simulink model "fourbar"  (Simulink 7.1)
settings: Solver=ode45  StartTime=0.0  StopTime=10  RelTol=1e-3
values from neighbouring files (symbols this model uses):
  m = 0    [FixNode1.m]    (also in FixNode2.m = xy(1,1)-x; SAM.m = str2num(char(m2))-str2num(char(m1)); angle_measurement.m = X(1,2)-X(1,1); m_645.m = 1)
  s = 0    [FixNode2.m]    (also in SAM.m = FixNode2(); linkm.m = -1.57079632679)
libraries: mblibv1 x15
settings Model: Creator=mohsen  LastModifiedBy=mohsen
settings SimMechanicsCC: VisOnUpdateDiagram=on  VisDuringSimulation=on

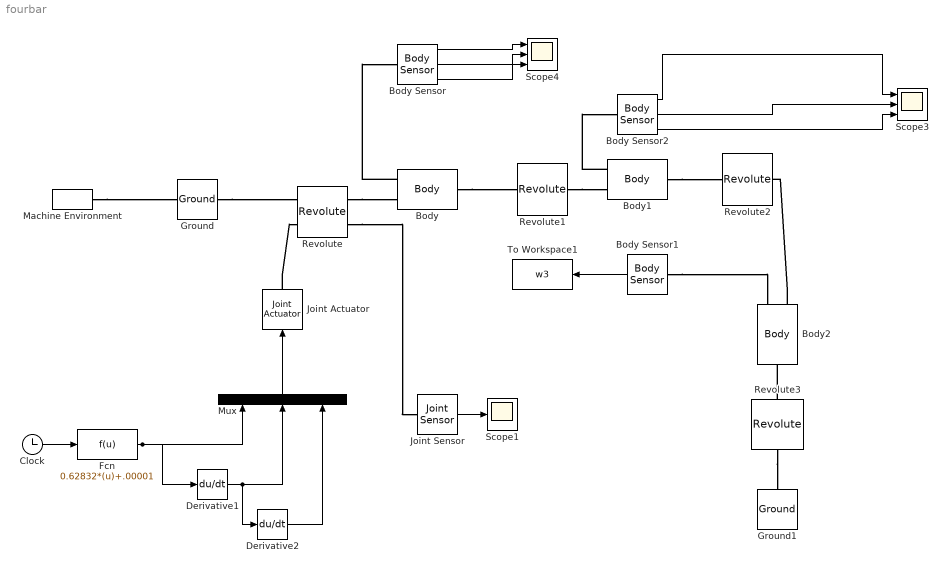
== system fourbar ==
  Body : mblibv1/Bodies/Body  DialogController=MECH.DynMechDlgSource  PhysicalDomain=mechanical  SubClassName=Unknown  LeftPortType=workingframe  RightPortType=workingframe  LConnTagsString=CS3|CS1  RConnTagsString=CS2  DialogClass=MechanicalBodyBlock  Mass=1  MassUnits=kg  InertiaUnits=kg*m^2  Inertia=[.1 0 0;0 .1 0;0 0 .1]  Shape=Cylinder  ShapeDims=[1 1]  ShapeUnits=m  ShapeUse=false  Density=1  DensityUnits=kg/m^3  DensityUse=false  GraphicsMode=1  BodyColor=[0.5 0.5 0.5]  GraphicsObj=[]  AttachedToCS=1  CG=Left$CG$[0 .5 0]$WORLD$WORLD$m$[0 0 0]$Euler X-Y-Z$deg$WORLD$false$none  WorkingFrames=Left$CS3$[0 .5 0]$WORLD$WORLD$m$[0 0 0]$Euler X-Y-Z$deg$WORLD$true$none#Left$CS1$[0 0 0]$World$World$m$[0 0 0]$Euler X-Y-Z$deg$WORLD$true$none#Right$CS2$[0 2 0]$World$World$m$[0 0 0]$Euler X-Y-Z$deg$WORLD$true$none  CGPos=[0 .5 0]  CGRot=[0 0 0]  CS0Pos=[]  CS0Rot=[]  CS1Pos=[0 0 0]  CS1Rot=[0 0 0]  CS2Pos=[0 2 0]  CS2Rot=[0 0 0]  CS3Pos=[0 .5 0]  CS3Rot=[0 0 0]  CS4Pos=[]  CS4Rot=[]  CS5Pos=[]  CS5Rot=[]  CS6Pos=[]  CS6Rot=[]  CS7Pos=[]  CS7Rot=[]  CS8Pos=[]  CS8Rot=[]  CS9Pos=[]  CS9Rot=[]  CS10Pos=[]  CS10Rot=[]  CS11Pos=[]  CS11Rot=[]  CS12Pos=[]  CS12Rot=[]  CS13Pos=[]  CS13Rot=[]  CS14Pos=[]  CS14Rot=[]  CS15Pos=[]  CS15Rot=[]  CS16Pos=[]  CS16Rot=[]  CS17Pos=[]  CS17Rot=[]  CS18Pos=[]  CS18Rot=[]  CS19Pos=[]  CS19Rot=[]  CS20Pos=[]  CS20Rot=[]
  Body Sensor : mblibv1/Sensors &  Actuators/Body Sensor  DialogController=MECH.DynMechDlgSource  SystemSampleTime=-1  PhysicalDomain=Mechanical  PortType=blob  Muxed=off  Pose=off  Angle=on  AngleUnits=deg  ArcVelocity=off  ArcVelocityUnits=deg/s  ArcAcceleration=off  ArcAccelerationUnits=deg/s^2  CoordPosition=on  CoordPositionUnits=m  Velocity=on  VelocityUnits=m/s  Acceleration=on  AccelerationUnits=m/s^2  Quaternion=on  QuaternionDT=off  QuaternionDDT=off  QuaternionUnits=off  OutputVector=[1]  ActiveIO=on  Width=9  DialogClass=MechanicalSensorBlock  ReferenceFrame=Absolute (World)
  Body Sensor1 : mblibv1/Sensors &  Actuators/Body Sensor  Orientation=left  DialogController=MECH.DynMechDlgSource  SystemSampleTime=-1  PhysicalDomain=Mechanical  PortType=blob  Muxed=on  Pose=off  Angle=on  AngleUnits=deg  ArcVelocity=off  ArcVelocityUnits=deg/s  ArcAcceleration=off  ArcAccelerationUnits=deg/s^2  CoordPosition=on  CoordPositionUnits=m  Velocity=off  VelocityUnits=m/s  Acceleration=off  AccelerationUnits=m/s^2  Quaternion=on  QuaternionDT=off  QuaternionDDT=off  QuaternionUnits=off  OutputVector=[1]  ActiveIO=on  Width=3  DialogClass=MechanicalSensorBlock  ReferenceFrame=Absolute (World)
  Body Sensor2 : mblibv1/Sensors &  Actuators/Body Sensor  DialogController=MECH.DynMechDlgSource  SystemSampleTime=-1  PhysicalDomain=Mechanical  PortType=blob  Muxed=off  Pose=off  Angle=on  AngleUnits=deg  ArcVelocity=off  ArcVelocityUnits=deg/s  ArcAcceleration=off  ArcAccelerationUnits=deg/s^2  CoordPosition=on  CoordPositionUnits=m  Velocity=on  VelocityUnits=m/s  Acceleration=on  AccelerationUnits=m/s^2  Quaternion=on  QuaternionDT=off  QuaternionDDT=off  QuaternionUnits=off  OutputVector=[1]  ActiveIO=on  Width=9  DialogClass=MechanicalSensorBlock  ReferenceFrame=Absolute (World)
  Body1 : mblibv1/Bodies/Body  DialogController=MECH.DynMechDlgSource  PhysicalDomain=mechanical  SubClassName=Unknown  LeftPortType=workingframe  RightPortType=workingframe  LConnTagsString=CS3|CS1  RConnTagsString=CS2  DialogClass=MechanicalBodyBlock  Mass=1  MassUnits=kg  InertiaUnits=kg*m^2  Inertia=[.1 0 0;0 .1 0;0 0 .1]  Shape=Cylinder  ShapeDims=[1 1]  ShapeUnits=m  ShapeUse=false  Density=1  DensityUnits=kg/m^3  DensityUse=false  GraphicsMode=1  BodyColor=[0.5 0.5 0.5]  GraphicsObj=[]  AttachedToCS=1  CG=Left$CG$[2 3 0]$WORLD$WORLD$m$[0 0 0]$Euler X-Y-Z$deg$WORLD$false$none  WorkingFrames=Left$CS3$[2 3 0]$WORLD$WORLD$m$[0 0 0]$Euler X-Y-Z$deg$WORLD$true$none#Left$CS1$[0 2 0]$World$World$m$[0 0 0]$Euler X-Y-Z$deg$WORLD$true$none#Right$CS2$[4 4 0]$World$World$m$[0 0 0]$Euler X-Y-Z$deg$WORLD$true$none  CGPos=[2 3 0]  CGRot=[0 0 0]  CS0Pos=[]  CS0Rot=[]  CS1Pos=[0 2 0]  CS1Rot=[0 0 0]  CS2Pos=[4 4 0]  CS2Rot=[0 0 0]  CS3Pos=[2 3 0]  CS3Rot=[0 0 0]  CS4Pos=[]  CS4Rot=[]  CS5Pos=[]  CS5Rot=[]  CS6Pos=[]  CS6Rot=[]  CS7Pos=[]  CS7Rot=[]  CS8Pos=[]  CS8Rot=[]  CS9Pos=[]  CS9Rot=[]  CS10Pos=[]  CS10Rot=[]  CS11Pos=[]  CS11Rot=[]  CS12Pos=[]  CS12Rot=[]  CS13Pos=[]  CS13Rot=[]  CS14Pos=[]  CS14Rot=[]  CS15Pos=[]  CS15Rot=[]  CS16Pos=[]  CS16Rot=[]  CS17Pos=[]  CS17Rot=[]  CS18Pos=[]  CS18Rot=[]  CS19Pos=[]  CS19Rot=[]  CS20Pos=[]  CS20Rot=[]
  Body2 : mblibv1/Bodies/Body  Orientation=down  DialogController=MECH.DynMechDlgSource  PhysicalDomain=mechanical  SubClassName=Unknown  LeftPortType=workingframe  RightPortType=workingframe  LConnTagsString=CS3|CS1  RConnTagsString=CS2  DialogClass=MechanicalBodyBlock  Mass=1  MassUnits=kg  InertiaUnits=kg*m^2  Inertia=[.1 0 0;0 .1 0;0 0 .1]  Shape=Cylinder  ShapeDims=[1 1]  ShapeUnits=m  ShapeUse=false  Density=1  DensityUnits=kg/m^3  DensityUse=false  GraphicsMode=1  BodyColor=[0.5 0.5 0.5]  GraphicsObj=[]  AttachedToCS=1  CG=Left$CG$[2.5 2 0]$WORLD$WORLD$m$[0 0 0]$Euler X-Y-Z$deg$WORLD$false$none  WorkingFrames=Left$CS3$[ 2.5 2 0]$WORLD$WORLD$m$[0 0 0]$Euler X-Y-Z$deg$WORLD$true$none#Left$CS1$[4 4 0]$World$World$m$[0 0 0]$Euler X-Y-Z$deg$WORLD$true$none#Right$CS2$[1 0 0]$World$World$m$[0 0 0]$Euler X-Y-Z$deg$WORLD$true$none  CGPos=[2.5 2 0]  CGRot=[0 0 0]  CS0Pos=[]  CS0Rot=[]  CS1Pos=[4 4 0]  CS1Rot=[0 0 0]  CS2Pos=[1 0 0]  CS2Rot=[0 0 0]  CS3Pos=[ 2.5 2 0]  CS3Rot=[0 0 0]  CS4Pos=[]  CS4Rot=[]  CS5Pos=[]  CS5Rot=[]  CS6Pos=[]  CS6Rot=[]  CS7Pos=[]  CS7Rot=[]  CS8Pos=[]  CS8Rot=[]  CS9Pos=[]  CS9Rot=[]  CS10Pos=[]  CS10Rot=[]  CS11Pos=[]  CS11Rot=[]  CS12Pos=[]  CS12Rot=[]  CS13Pos=[]  CS13Rot=[]  CS14Pos=[]  CS14Rot=[]  CS15Pos=[]  CS15Rot=[]  CS16Pos=[]  CS16Rot=[]  CS17Pos=[]  CS17Rot=[]  CS18Pos=[]  CS18Rot=[]  CS19Pos=[]  CS19Rot=[]  CS20Pos=[]  CS20Rot=[]
  Clock : Clock
      settings: Decimation=10
  Derivative1 : Derivative
  Derivative2 : Derivative
  Fcn : Fcn  Expr=0.62832*(u)+.00001
      settings: AttributesFormatString=%<Expr>
  Ground : mblibv1/Bodies/Ground  DialogController=MECH.DynMechDlgSource  SystemSampleTime=-1  LeftPortType=env  RightPortType=workingframe  PhysicalDomain=Mechanical  DialogClass=GroundBlock  CoordPosition=[0 0 0]  CoordPositionUnits=m  StateVectorMgrId=6  MachineId=[7 0]  ShowEnvPort=on
  Ground1 : mblibv1/Bodies/Ground  Orientation=up  DialogController=MECH.DynMechDlgSource  SystemSampleTime=-1  LeftPortType=env  RightPortType=workingframe  PhysicalDomain=Mechanical  DialogClass=GroundBlock  CoordPosition=[1 0 0]  CoordPositionUnits=m  StateVectorMgrId=-1  MachineId=[0 0]  ShowEnvPort=off
  Joint Actuator : mblibv1/Sensors &  Actuators/Joint Actuator  Orientation=up  DialogController=MECH.DynMechDlgSource  SystemSampleTime=-1  PhysicalDomain=Mechanical  PortType=blob  ActuationStyle=Motion  AngleUnits=rad  ArcVelocityUnits=rad/s  ArcAccelerationUnits=rad/s^2  CoordPositionUnits=m  VelocityUnits=m/s  AccelerationUnits=m/s^2  ForceUnits=N  TorqueUnits=N*m  ActiveIO=on  Width=3  DialogClass=MechanicalActuatorBlock  Primitive=R1  ReferenceFrame=Absolute (World)
  Joint Sensor : mblibv1/Sensors &  Actuators/Joint Sensor  DialogController=MECH.DynMechDlgSource  SystemSampleTime=-1  PhysicalDomain=Mechanical  PortType=blob  Muxed=on  Pose=off  Angle=off  AngleUnits=deg  ArcVelocity=on  ArcVelocityUnits=deg/s  ArcAcceleration=off  ArcAccelerationUnits=deg/s^2  CoordPosition=on  CoordPositionUnits=m  Velocity=off  VelocityUnits=m/s  Acceleration=off  AccelerationUnits=m/s^2  Quaternion=on  QuaternionDT=off  QuaternionDDT=off  QuaternionUnits=off  OutputVector=[1]  ActiveIO=on  Width=1  DialogClass=MechanicalSensorBlock  Primitive=R1  Force=off  ForceUnits=N  Torque=off  TorqueUnits=N*m  ReferenceFrame=Absolute (World)  ReactionSensedSide=Base  ReactionReferenceFrame=Absolute (World)  ReactionForce=off  ReactionForceUnits=N  ReactionMoment=off  ReactionMomentUnits=N*m
  Machine Environment : mblibv1/Bodies/Machine Environment  DialogController=MECH.DialogSource  SystemSampleTime=-1  PortType=env  PhysicalDomain=Mechanical  DialogTemplateClass=MECH.MachineEnvironment  SyncWhenCopied=off  Gravity=[0 -9.81 0]  GravityUnits=m/s^2  GravityAsSignal=off  Dimensionality=Auto-detect  AnalysisType=Forward dynamics  LinearAssemblyTolerance=1e-3  LinearAssemblyToleranceUnits=m  AngularAssemblyTolerance=1e-3  AngularAssemblyToleranceUnits=rad  ConstraintSolverType=Stabilizing  ConstraintRelTolerance=1e-4  ConstraintAbsTolerance=1e-4  UseRobustSingularityHandling=off  RedundancyAnalysisToleranceType=Automatically select tolerance  RedundancyAnalysisTolerance=1e-14  StatePerturbationType=Fixed  PerturbationSize=1e-5  VisualizeMachine=on
  Mux : Mux  Orientation=up  Inputs=3
  Revolute : mblibv1/Joints/Revolute  DialogController=MECH.DynMechDlgSource  PhysicalDomain=mechanical  SubClassName=Unknown  LeftPortType=blob  RightPortType=blob  LConnTagsString=__newl0|SA1  RConnTagsString=__newr0|SA1  NumSAPorts=2  CutJoint=off  MarkAsCut=off  Primitives=prismatic  PrimitiveProps=R1$World$[0 0 1]$revolute  DialogClass=JointBlock  R1Axis=[0 0 1]
  Revolute1 : mblibv1/Joints/Revolute  DialogController=MECH.DynMechDlgSource  PhysicalDomain=mechanical  SubClassName=Unknown  LeftPortType=blob  RightPortType=blob  LConnTagsString=__newl0  RConnTagsString=__newr0  NumSAPorts=0  CutJoint=off  MarkAsCut=off  Primitives=prismatic  PrimitiveProps=R1$World$[0 0 1]$revolute  DialogClass=JointBlock  R1Axis=[0 0 1]
  Revolute2 : mblibv1/Joints/Revolute  DialogController=MECH.DynMechDlgSource  PhysicalDomain=mechanical  SubClassName=Unknown  LeftPortType=blob  RightPortType=blob  LConnTagsString=__newl0  RConnTagsString=__newr0  NumSAPorts=0  CutJoint=off  MarkAsCut=off  Primitives=prismatic  PrimitiveProps=R1$World$[0 0 1]$revolute  DialogClass=JointBlock  R1Axis=[0 0 1]
  Revolute3 : mblibv1/Joints/Revolute  Orientation=down  DialogController=MECH.DynMechDlgSource  PhysicalDomain=mechanical  SubClassName=Unknown  LeftPortType=blob  RightPortType=blob  LConnTagsString=__newl0  RConnTagsString=__newr0  NumSAPorts=0  CutJoint=off  MarkAsCut=off  Primitives=prismatic  PrimitiveProps=R1$World$[0 0 1]$revolute  DialogClass=JointBlock  R1Axis=[0 0 1]
  Scope1 : Scope
  Scope3 : Scope  NumInputPorts=3
      settings: YMin=-5~-5~-5  YMax=5~5~5  SaveName=ScopeData3
  Scope4 : Scope  NumInputPorts=3
      settings: YMin=-5~-5~-5  YMax=5~5~5  SaveName=ScopeData4
  To Workspace1 : ToWorkspace  VariableName=w3  SampleTime=-1  SaveFormat=Structure With Time
  wires:
  Mux/1 -> Joint Actuator/1
  Body Sensor1/1 -> To Workspace1/1
  Joint Sensor/1 -> Scope1/1
  Fcn/1 -> Derivative1/1, Mux/1
  Derivative1/1 -> Mux/2, Derivative2/1
  Derivative2/1 -> Mux/3
  Clock/1 -> Fcn/1
  Body Sensor/1 -> Scope4/1
  Body Sensor/2 -> Scope4/2
  Body Sensor2/1 -> Scope3/1
  Body Sensor2/2 -> Scope3/2
  Body Sensor2/3 -> Scope3/3
  Body Sensor/3 -> Scope4/3
  connections:
  Revolute3/LConn1 -- Body2/RConn1
  Body2/LConn2 -- Revolute2/RConn1
  Machine Environment/RConn1 -- Ground/LConn1
  Ground/RConn1 -- Revolute/LConn1
  Revolute/RConn2 -- Joint Sensor/LConn1
  Revolute/RConn1 -- Body/LConn2
  Revolute1/RConn1 -- Body1/LConn2
  Body/LConn1 -- Body Sensor/LConn1
  Body Sensor1/LConn1 -- Body2/LConn1
  Body/RConn1 -- Revolute1/LConn1
  Revolute3/RConn1 -- Ground1/RConn1
  Body1/RConn1 -- Revolute2/LConn1
  Joint Actuator/RConn1 -- Revolute/LConn2
  Body1/LConn1 -- Body Sensor2/LConn1
